simulink model "dbg2"  (R2018a)
settings: Solver=VariableStepAuto  StartTime=0.0  StopTime=70  MaxStep=1e-2  RelTol=1e-3
values from neighbouring files (symbols this model uses):
  b = 2    [sp.m]
  b1 = 1    [sp.m]
  D2 = 1    [sp.m]
  J = 3    [sp.m]
  J1 = 3    [sp.m]
  k = 3    [sp.m]
  M = 2    [sp.m]
  N1 = 10    [sp.m]
  N2 = 20    [sp.m]
  N3 = 30    [sp.m]
  N4 = 60    [sp.m]
  R = 2    [sp.m]
  T = 2    [sp.m]
settings Model: Creator=carma  LastModifiedBy=carma

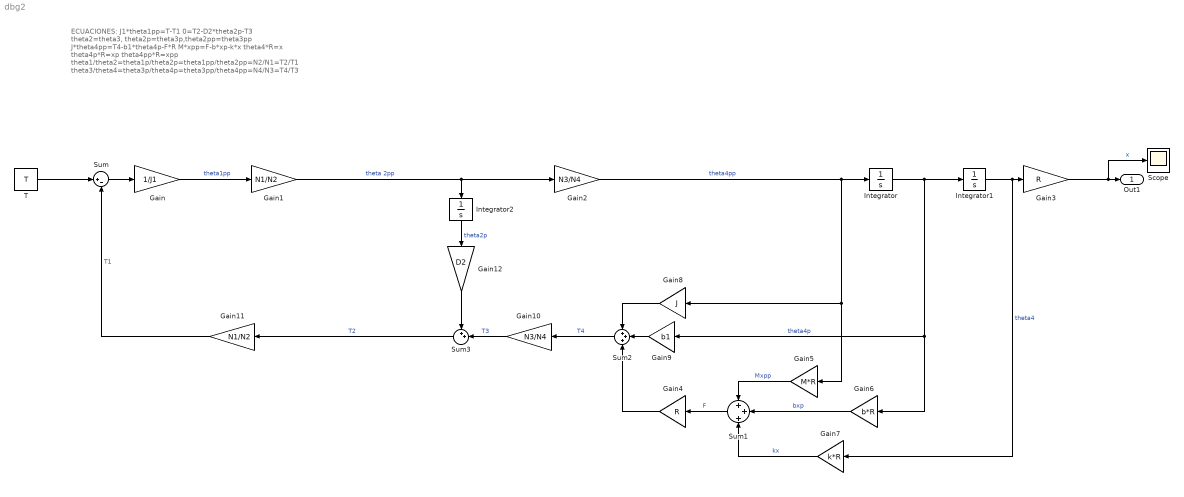
== system dbg2 ==
  note: ECUACIONES:
      | J1*theta1pp=T-T1
      | 0=T2-D2*theta2p-T3
      | theta2=theta3, theta2p=theta3p,theta2pp=theta3pp
      | J*theta4pp=T4-b1*theta4p-F*R
      | M*xpp=F-b*xp-k*x
      | theta4*R=x theta4p*R=xp theta4pp*R=xpp
      | theta1/theta2=theta1p/theta2p=theta1pp/theta2pp=N2/N1=T2/T1
      | theta3/theta4=theta3p/theta4p=theta3pp/theta4pp=N4/N3=T4/T3
  Gain : Gain  Gain=1/J1
  Gain1 : Gain  Gain=N1/N2
  Gain10 : Gain  Gain=N3/N4
  Gain11 : Gain  Gain=N1/N2
  Gain12 : Gain  Gain=D2
  Gain2 : Gain  Gain=N3/N4
  Gain3 : Gain  Gain=R
  Gain4 : Gain  Gain=R
  Gain5 : Gain  Gain=M*R
  Gain6 : Gain  Gain=b*R
  Gain7 : Gain  Gain=k*R
  Gain8 : Gain  Gain=J
  Gain9 : Gain  Gain=b1
  Integrator : Integrator
  Integrator1 : Integrator
  Integrator2 : Integrator
  Scope : Scope
  Sum : Sum  Inputs=|+-
  Sum1 : Sum  Inputs=+++
  Sum2 : Sum  Inputs=+++
  Sum3 : Sum  Inputs=++|
  T : Constant  Value=T
  Out1 : Outport
  wires:
  T/1 -> Sum/1
  Sum/1 -> Gain/1
  Integrator/1 -> Gain9/1, Gain6/1, Integrator1/1  "theta4p"
  Gain/1 -> Gain1/1  "theta1pp"
  Gain1/1 -> Integrator2/1, Gain2/1  "theta 2pp"
  Gain2/1 -> Gain5/1, Gain8/1, Integrator/1  "theta4pp"
  Integrator1/1 -> Gain7/1, Gain3/1  "theta4"
  Gain3/1 -> Scope/1, Out1/1  "x"
  Gain5/1 -> Sum1/1  "Mxpp"
  Sum1/1 -> Gain4/1  "F"
  Gain6/1 -> Sum1/2  "bxp"
  Gain7/1 -> Sum1/3  "kx"
  Gain8/1 -> Sum2/1
  Gain4/1 -> Sum2/3
  Gain9/1 -> Sum2/2
  Sum2/1 -> Gain10/1  "T4"
  Gain11/1 -> Sum/2  "T1"
  Gain10/1 -> Sum3/2  "T3"
  Integrator2/1 -> Gain12/1  "theta2p"
  Sum3/1 -> Gain11/1  "T2"
  Gain12/1 -> Sum3/1
